simulink model "sub"  (R2018a)
settings: Solver=FixedStepAuto  StartTime=0.0  StopTime=0.00004  RelTol=1e-3  EnableMultiTasking=on
InitFcn:
  | %% DSPBuilder Start
  | alt_dspbuilder_update_model(bdroot)
  | %% DSPBuilder End
StartFcn:
  | %% DSPBuilder Start
  | alt_dspbuilder_hdlimport_prepare_for_simulation(bdroot)
  | %% DSPBuilder End
libraries: allblocks_alteradspbuilder2 x6, dspsigops x1
settings Model: Creator=klutc_000  LastModifiedBy=klutc_000
settings SolverCC: AutoInsertRateTranBlk=on
settings DebuggingCC: SingleTaskRateTransMsg=error

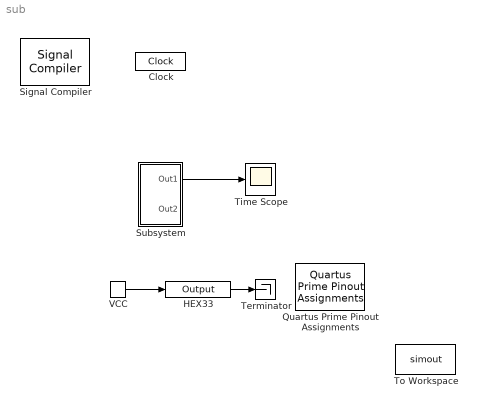
== system sub ==
  Clock : allblocks_alteradspbuilder2/Clock  ClockPeriod=20  ClockPeriodUnit=ns  SampleTime=1/50000000  ResetLatency=0  ResetRegisterCascadeDepth=0  SimulationStartCycle=5  PhaseOffset=0  Reset=aclr  ResetType=Active Low  Export=off
  HEX33 : allblocks_alteradspbuilder2/Output  iofile=D:\dspb_serum\tb_sub\sub_HEX33.capture  BusType=Single Bit  bwl=1  bwr=0  externalType=Inferred  PORTTYPE=Output  allowFloatingPointOverride=on  logOutputs=off
  Quartus Prime Pinout Assignments : allblocks_alteradspbuilder2/Quartus Prime Pinout Assignments  QuartusIIAssignmentName=HEX33  QuartusIIAssignmentValue=PIN_E4
  Signal Compiler : allblocks_alteradspbuilder2/Signal Compiler  DeviceFamily=Cyclone IV GX  DeviceName=AUTO  DisableEarlyHDLGeneration=off  EnableSignalTap=off  SignalTapDepth=128  UseBoardBlock=off  StpUseDefaultClock=on  StpClock=Clock  ExportDir=D:\intelFPGA\16.1\quartus\dsp_builder  MAX10_ProgrammingMode=Internal Flash (SDM) Single Boot
  Subsystem : Subsystem
  Terminator : Terminator
  Time Scope : Scope
  To Workspace : ToWorkspace  VariableName=simout  SampleTime=-1
      settings: Save2DSignal=2-D array (concatenate along first dimension)
  VCC : allblocks_alteradspbuilder2/VCC  SpecifyClock=off
  wires:
  Subsystem/1(Out1) -> Time Scope/1
  VCC/1 -> HEX33/1
  HEX33/1 -> Terminator/1

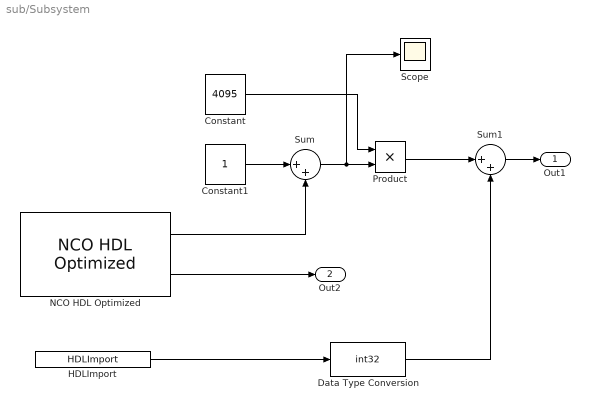
== system sub/Subsystem ==
  Constant : Constant  Value=4095  VectorParams1D=off  OutDataTypeStr=double  SampleTime=-1
  Constant1 : Constant  VectorParams1D=off  OutDataTypeStr=double  SampleTime=-1
  Data Type Conversion : DataTypeConversion  OutDataTypeStr=int32
  HDLImport : allblocks_alteradspbuilder2/HDLImport  entityName=trigen_import  outNames=triout  outBwls=32  outBwrs=0  outTypes=s  xmlmapfile=D:\intelFPGA\16.1\quartus\dsp_builder\lib\SimgenCMap.xml  vofile=DSPBuilder_tmod_import\trigen.vo  src_file=hdl_prj\hdlsrc\tmod\trigen.vhd;  TopLevelName=trigen  UseQPF=0  n_input_port=0  n_output_port=1  array_clocks=clock  use_systemC_model=off  is_megacore=off  use_dynamic_feedthrough_data=off  use_alphabetical_port_ordering=on  allowFloatingPointOverride=off  id=0  id_is_set=off  UseModelSimBasedFlow=off
  NCO HDL Optimized : dspsigops/NCO HDL Optimized  PhaseIncrementSource=Property  PhaseIncrement=100  PhaseOffsetSource=Property  PhaseOffset=0  DitherSource=Property  NumDitherBits=4  PhaseQuantization=on  NumQuantizerAccumulatorBits=12  LUTCompress=off  ResetAction=off  ValidInputPort=off  Waveform=Sine  PhasePort=off  SimulateUsing=Code generation  AccumulatorWL=16  OutputDataType=double  OutputWL=32  OutputFL=2
      settings: SourceProductName=DSP System Toolbox  SourceProductBaseCode=DS
  Product : Product  OutDataTypeStr=int32
  Scope : Scope
  Sum : Sum  Inputs=|++  OutDataTypeStr=double
  Sum1 : Sum  Inputs=|++  OutDataTypeStr=int32
  Out1 : Outport
  Out2 : Outport  Port=2
  wires:
  HDLImport/1 -> Data Type Conversion/1
  Constant/1 -> Product/1
  NCO HDL Optimized/2 -> Out2/1
  Constant1/1 -> Sum/1
  NCO HDL Optimized/1 -> Sum/2
  Sum/1 -> Scope/1, Product/2
  Product/1 -> Sum1/1
  Data Type Conversion/1 -> Sum1/2
  Sum1/1 -> Out1/1
